simulink model "Li_Slotine"  (R2021b)
settings: Solver=VariableStepAuto  StartTime=0.0  StopTime=15.0  FixedStep=1e-3  MaxStep=1e-1  RelTol=1e1
values from neighbouring files (symbols this model uses):
  Kd = diag([100 500 300 100 1 1])    [GuadagniControllore.m]    (also in LS_workspace.mat = [100 0 0 0 0 0 0 500 0 0 0 0 ... (36 elements, 6x6)])
  l1 = 0.1273    [LS_workspace.mat]
  l2 = -0.612    [LS_workspace.mat]
  l3 = -0.5723    [LS_workspace.mat]
  l4 = 0.1639    [LS_workspace.mat]
  l5 = 0.1157    [LS_workspace.mat]
  l6 = 0.0922    [LS_workspace.mat]
  lambda = diag([20 100 80 36 50 100])    [GuadagniControllore.m]    (also in LS_workspace.mat = [20 0 0 0 0 0 0 100 0 0 0 0 ... (36 elements, 6x6)])
  m1 = L(1).m    [GuadagniControllore.m]    (also in LS_workspace.mat = 7.1)
  m2 = L(2).m    [GuadagniControllore.m]    (also in LS_workspace.mat = 12.7)
  m3 = L(3).m    [GuadagniControllore.m]    (also in LS_workspace.mat = 4.27)
  m4 = L(4).m    [GuadagniControllore.m]    (also in LS_workspace.mat = 2)
  m5 = L(5).m    [GuadagniControllore.m]    (also in LS_workspace.mat = 2)
  m6 = L(6).m    [GuadagniControllore.m]    (also in LS_workspace.mat = 0.365)
  Q_des = [-2.30401536147 -2.31146826059 -2.31936116359 -2.32763094017 -2.33621351701 -2.34504499078 -2.35406266963 -2.36320601211 -2.3724174398 -2.38164300799 -2.3908329269 -2.3999419333 ... (3000 elements, 500x6)]    [LS_workspace.mat]
  r = 0.02    [LS_workspace.mat]
undefined symbols (not defined in the file or in its folder): B, Spline
libraries: roblocks x2, robotcorelib x1, simulink x1
(part 5 of 5)

== matlab function Li_Slotine/Li-Slotine control/parameters estimation ==
  data: Y input; dpi output; s input
function dpi = dyn_param(Y, s)
% Definisco una matrice definita positiva
R = diag([0.1382 22 145 240 250 1490]);
% Calcolo la dinamica di stima dei parametri
dpi = inv(R) * Y' * s;

== matlab function Li_Slotine/Li-Slotine control/MATLAB Function ==
  data: e input; qr_d output; e_dot input; qd_des input; qdd_des input; qr_dd output; lambda input
function [qr_d, qr_dd] = qr_d_calculus(e, e_dot, qd_des, qdd_des, lambda)
% Calcolo qr_d
qr_d = qd_des + lambda*e;
% Calcolo qr_dd
qr_dd = qdd_des + lambda*e_dot;
